simulink model "OFDM_64QAM_R14"  (Simulink 10.0)
settings: Solver=VariableStepDiscrete  StartTime=0.0  StopTime=5000  RelTol=1e-3  EnableMultiTasking=on
undefined symbols (not defined in the file): get
libraries: commutil2 x4, commsink2 x3, commdigbbndam2 x2, dspxfrm3 x2, dspindex x2, dspbuff3 x2, dspsnks4 x2, commchan2 x1, commrandsrc2 x1, dspobslib x1, simulink x1
settings Model: Creator=khanm  LastModifiedBy=bhisma
settings DataIOCC: ExternalInput=input_data  LimitDataPoints=on  SignalLoggingSaveFormat=ModelDataLogs  SaveOutput=off  SignalLogging=off  SaveTime=off
settings OptimizationCC: ExpressionDepthLimit=2147483647  InitFltsAndDblsToZero=on
settings DebuggingCC: SaveWithParameterizedLinksMsg=none  SignalResolutionControl=TryResolveAllWithWarning  MultiTaskDSMMsg=warning  MultiTaskCondExecSysMsg=none  FcnCallInpInsideContextMsg=warning  StateNameClashWarn=warning
settings SFSimCC: SimUseLocalCustomCode=on  CustomCodeUndefinedFunction=FilterOut
settings RTWCC: RTWUseLocalCustomCode=on
settings GRTTargetCC: TargetFcnLib=ansi_tfl_tmw.mat

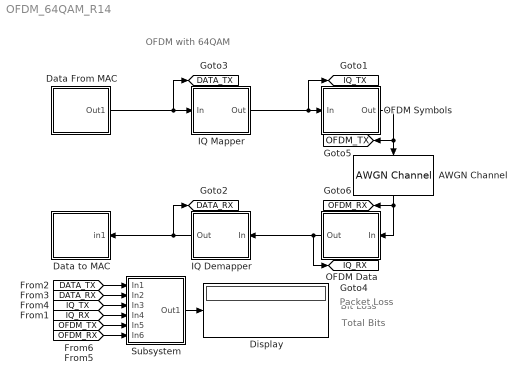
== system OFDM_64QAM_R14 ==
  note: OFDM with 64QAM
  note: Total Bits
  note: Bit Loss
  note: Packet Loss
  AWGN Channel : commchan2/AWGN Channel  SystemSampleTime=-1  seed=1  noiseMode="Signal to noise ratio  (SNR)"  EbNodB=10  EsNodB=40  SNRdB=60  bitsPerSym=2  Ps=0.01  Tsym=4e-6/80  variance=1
      settings: SourceProductName=Communications Toolbox  SourceProductBaseCode=CM
  Data From MAC : Subsystem
      mask Display: disp('Data Source');
  Data to MAC : Subsystem
      mask Display: disp('Data Sink');
  Display : Display
  IQ Demapper : Subsystem
      mask Display: disp('IQ Demapper');
  IQ Mapper : Subsystem
      mask Display: disp('IQ Mapper');
  OFDM Data : Subsystem
      mask Display: disp('OFDM \n Demodulator');
  OFDM Symbols : Subsystem
      mask Display: disp(' OFDM \n Modulation');
  Subsystem : Subsystem
      mask Display: disp('System\nPerformance\nTests');
  tag scope: DATA_RX=global, DATA_TX=global, IQ_RX=global, IQ_TX=global, OFDM_RX=global, OFDM_TX=global
  wires:
  IQ Demapper/1(Out) -> Data to MAC/1(in1), [DATA_RX]
  AWGN Channel/1 -> OFDM Data/1(In), [OFDM_RX]
  OFDM Data/1(Out) -> IQ Demapper/1(In), [IQ_RX]
  OFDM Symbols/1(Out) -> AWGN Channel/1, [OFDM_TX]
  IQ Mapper/1(Out) -> OFDM Symbols/1(In), [IQ_TX]
  [DATA_TX] -> Subsystem/1(In1)
  [DATA_RX] -> Subsystem/2(In2)
  [IQ_TX] -> Subsystem/3(In3)
  [IQ_RX] -> Subsystem/4(In4)
  [OFDM_TX] -> Subsystem/5(In5)
  [OFDM_RX] -> Subsystem/6(In6)
  Subsystem/1(Out1) -> Display/1
  Data From MAC/1(Out1) -> IQ Mapper/1(In), [DATA_TX]

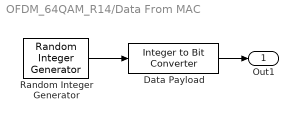
== system OFDM_64QAM_R14/Data From MAC ==
  Data Payload : commutil2/Integer to Bit Converter  nbits=6
      settings: SourceProductName=Communications Toolbox
  Random Integer Generator : commrandsrc2/Random Integer Generator  SystemSampleTime=-1  mul=32  seed=37  Ts=1/192  frameBased=on  sampPerFrame=192  orient=off
      settings: SourceProductName=Communications Toolbox  SourceProductBaseCode=CM
  Out1 : Outport
  wires:
  Random Integer Generator/1 -> Data Payload/1
  Data Payload/1 -> Out1/1

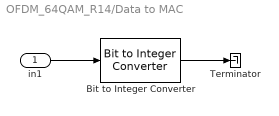
== system OFDM_64QAM_R14/Data to MAC ==
  in1 : Inport
  Bit to Integer Converter : commutil2/Bit to Integer Converter  nbits=6
      settings: SourceProductName=Communications Toolbox
  Terminator : Terminator
  wires:
  in1/1 -> Bit to Integer Converter/1
  Bit to Integer Converter/1 -> Terminator/1

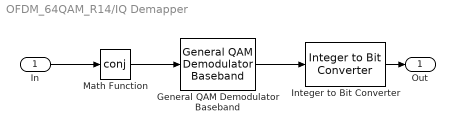
== system OFDM_64QAM_R14/IQ Demapper ==
  In : Inport
  General QAM Demodulator Baseband : commdigbbndam2/General QAM Demodulator Baseband  SigCon="[0.4629 + 0.4629i    0.4629 + 0.1543i    0.4629 + 0.7715i    0.4629 + 1.0801i    0.4629 - 0.4629i    0.4629 - 0.1543i    0.4629 - 0.7715i    0.4629 - 1.0801i    0.1543 + 0.4629i    0.1543 + 0.1543i    0.1543 + 0.7715i    0.1543 + 1.0801i    0.1543 - 0.4629i    0.1543 - 0.1543i    0.1543 - 0.7715i    0.1543 - 1.0801i    0.7715 + 0.4629i    0.7715 + 0.1543i    0.7715 + 0.7715i    0.7715 + 1.0801i    0.7715 - 0.4629i    0.7715 - 0.1543i    0.7715 - 0.7715i    0.7715 - 1.0801i    1.0801 + 0.4629i    1.0801 + 0.1543i    1.0801 + 0.7715i    1.0801 + 1.0801i    1.0801 - 0.4629i    1.0801 - 0.1543i    1.0801 - 0.7715i    1.0801 - 1.0801i   -0.4629 + 0.4629i   -0.4629 + 0.1543i   -0.4629 + 0.7715i   -0.4629 + 1.0801i   -0.4629 - 0.4629i   -0.4629 - 0.1543i   -0.4629 - 0.7715i   -0.4629 - 1.0801i   -0.1543 + 0.4629i   -0.1543 + 0.1543i   -0.1543 + 0.7715i   -0.1543 + 1.0801i   -0.1543 - 0.4629i   -0.1543 - 0.1543i   -0.1543 - 0.7715i   -0.1543 - 1.0801i   -0.7715 + 0.4629i   -0.7715 + 0.1543i   -0.7715 + 0.7715i   -0.7715 + 1.0801i   -0.7715 - 0.4629i   -0.7715 - 0.1543i   -0.7715 - 0.7715i   -0.7715 - 1.0801i   -1.0801 + 0.4629i   -1.0801 + 0.1543i   -1.0801 + 0.7715i   -1.0801 + 1.0801i   -1.0801 - 0.4629i   -1.0801 - 0.1543i   -1.0801 - 0.7715i   -1.0801 - 1.0801i]'"  numSamp=1
  Integer to Bit Converter : commutil2/Integer to Bit Converter  nbits=6
      settings: SourceProductName=Communications Toolbox
  Math Function : Math  Operator=conj  SaturateOnIntegerOverflow=on
  Out : Outport
  wires:
  General QAM Demodulator Baseband/1 -> Integer to Bit Converter/1
  In/1 -> Math Function/1
  Math Function/1 -> General QAM Demodulator Baseband/1
  Integer to Bit Converter/1 -> Out/1

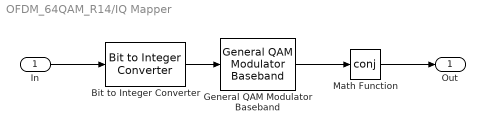
== system OFDM_64QAM_R14/IQ Mapper ==
  In : Inport
  Bit to Integer Converter : commutil2/Bit to Integer Converter  nbits=6
      settings: SourceProductName=Communications Toolbox
  General QAM Modulator Baseband : commdigbbndam2/General QAM Modulator Baseband  SigCon="[0.4629 + 0.4629i    0.4629 + 0.1543i    0.4629 + 0.7715i    0.4629 + 1.0801i    0.4629 - 0.4629i    0.4629 - 0.1543i    0.4629 - 0.7715i    0.4629 - 1.0801i    0.1543 + 0.4629i    0.1543 + 0.1543i    0.1543 + 0.7715i    0.1543 + 1.0801i    0.1543 - 0.4629i    0.1543 - 0.1543i    0.1543 - 0.7715i    0.1543 - 1.0801i    0.7715 + 0.4629i    0.7715 + 0.1543i    0.7715 + 0.7715i    0.7715 + 1.0801i    0.7715 - 0.4629i    0.7715 - 0.1543i    0.7715 - 0.7715i    0.7715 - 1.0801i    1.0801 + 0.4629i    1.0801 + 0.1543i    1.0801 + 0.7715i    1.0801 + 1.0801i    1.0801 - 0.4629i    1.0801 - 0.1543i    1.0801 - 0.7715i    1.0801 - 1.0801i   -0.4629 + 0.4629i   -0.4629 + 0.1543i   -0.4629 + 0.7715i   -0.4629 + 1.0801i   -0.4629 - 0.4629i   -0.4629 - 0.1543i   -0.4629 - 0.7715i   -0.4629 - 1.0801i   -0.1543 + 0.4629i   -0.1543 + 0.1543i   -0.1543 + 0.7715i   -0.1543 + 1.0801i   -0.1543 - 0.4629i   -0.1543 - 0.1543i   -0.1543 - 0.7715i   -0.1543 - 1.0801i   -0.7715 + 0.4629i   -0.7715 + 0.1543i   -0.7715 + 0.7715i   -0.7715 + 1.0801i   -0.7715 - 0.4629i   -0.7715 - 0.1543i   -0.7715 - 0.7715i   -0.7715 - 1.0801i   -1.0801 + 0.4629i   -1.0801 + 0.1543i   -1.0801 + 0.7715i   -1.0801 + 1.0801i   -1.0801 - 0.4629i   -1.0801 - 0.1543i   -1.0801 - 0.7715i   -1.0801 - 1.0801i]'"  numSamp=1
  Math Function : Math  Operator=conj  SaturateOnIntegerOverflow=on
  Out : Outport
  wires:
  In/1 -> Bit to Integer Converter/1
  General QAM Modulator Baseband/1 -> Math Function/1
  Math Function/1 -> Out/1
  Bit to Integer Converter/1 -> General QAM Modulator Baseband/1

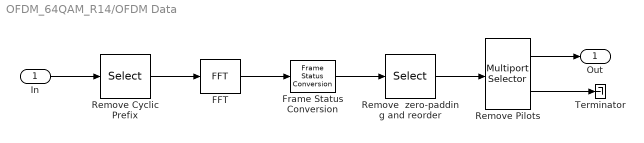
== system OFDM_64QAM_R14/OFDM Data ==
  In : Inport
  FFT : dspxfrm3/FFT  CompMethod=Table lookup  TableOpt=Speed  BitRevOrder=off  InheritFFTLength=on  FFTLength=64  SkipNorm=on  roundingMode=Floor  overflowMode=off
  Frame Status Conversion : dspobslib/Frame Status Conversion  SystemSampleTime=-1  growRefPort=off  outframe=Frame-based
      settings: SourceProductName=DSP System Toolbox  SourceProductBaseCode=DS
  Remove  zero-padding and reorder : Selector  InputPortWidth=256  IndexOptions=Index vector (dialog)  Indices=[29:128 130:229]  OutputSizes=[(-2)]
  Remove Pilots : dspindex/Multiport Selector  rowsOrCols=Rows  idxCellArray={[1:12 14:37 39:62 64:87 89:112 114:137 139:162 164:187 189:200],[13 38 63 88 113 138 163 188]}  idxErrMode=Clip Index
  Remove Cyclic Prefix : Selector  InputPortWidth=320  IndexOptions=Index vector (dialog)  Indices=[65:320]  OutputSizes=[(-2)]
  Terminator : Terminator
  Out : Outport
  wires:
  Frame Status Conversion/1 -> Remove  zero-padding and reorder/1
  FFT/1 -> Frame Status Conversion/1
  In/1 -> Remove Cyclic Prefix/1
  Remove  zero-padding and reorder/1 -> Remove Pilots/1
  Remove Pilots/1 -> Out/1
  Remove Pilots/2 -> Terminator/1
  Remove Cyclic Prefix/1 -> FFT/1

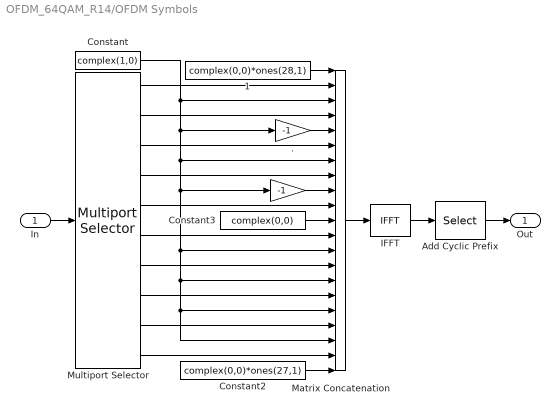
== system OFDM_64QAM_R14/OFDM Symbols ==
  In : Inport
  " " : Gain  Gain=-1
  " 1" : Constant  Value=complex(0,0)*ones(28,1)
  . : Gain  Gain=-1
  Add Cyclic Prefix : Selector  InputPortWidth=256  IndexOptions=Index vector (dialog)  Indices=[193:256 1:256]  OutputSizes=[(-2)]
  Constant : Constant  Value=complex(1,0)
  Constant2 : Constant  Value=complex(0,0)*ones(27,1)
  Constant3 : Constant  Value=complex(0,0)
  IFFT : dspxfrm3/IFFT  CompMethod=Table lookup  TableOpt=Speed  BitRevOrder=off  cs_in=off  SkipNorm=off  InheritFFTLength=on  FFTLength=64  mode=Complex  roundingMode=Floor  overflowMode=off
      settings: SourceProductName=DSP System Toolbox
  Matrix Concatenation : simulink/Math Operations/Matrix Concatenation  numInports=21  catMethod=Vertical
      settings: SourceProductName=Simulink  SourceProductBaseCode=SL
  Multiport Selector : dspindex/Multiport Selector  rowsOrCols=Rows  idxCellArray={1:12, 13:36, 37:60, 61:84, 85:96, 97:108, 109:132, 133:156, 157:180, 181:192}  idxErrMode=Clip Index
  Out : Outport
  wires:
  In/1 -> Multiport Selector/1
  Multiport Selector/9 -> Matrix Concatenation/18
  Multiport Selector/8 -> Matrix Concatenation/16
  Multiport Selector/7 -> Matrix Concatenation/14
  Multiport Selector/6 -> Matrix Concatenation/12
  Multiport Selector/5 -> Matrix Concatenation/10
  Multiport Selector/4 -> Matrix Concatenation/8
  Multiport Selector/3 -> Matrix Concatenation/6
  Multiport Selector/2 -> Matrix Concatenation/4
  Multiport Selector/1 -> Matrix Concatenation/2
  Multiport Selector/10 -> Matrix Concatenation/20
  Constant/1 -> Matrix Concatenation/3, Matrix Concatenation/7, " "/1, Matrix Concatenation/13, Matrix Concatenation/15, Matrix Concatenation/19, Matrix Concatenation/17, ./1
  " 1"/1 -> Matrix Concatenation/1
  Constant2/1 -> Matrix Concatenation/21
  ./1 -> Matrix Concatenation/5
  " "/1 -> Matrix Concatenation/9
  Constant3/1 -> Matrix Concatenation/11
  IFFT/1 -> Add Cyclic Prefix/1
  Matrix Concatenation/1 -> IFFT/1
  Add Cyclic Prefix/1 -> Out/1

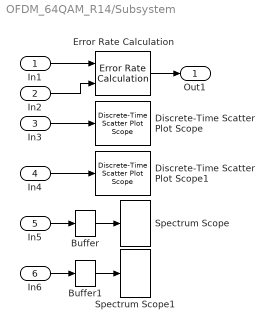
== system OFDM_64QAM_R14/Subsystem ==
  In1 : Inport
  In2 : Inport  Port=2
  In3 : Inport  Port=3
  In4 : Inport  Port=4
  In5 : Inport  Port=5
  In6 : Inport  Port=6
  Buffer : dspbuff3/Buffer  N=256  V=0  ic=0
      settings: SourceProductName=DSP System Toolbox  SourceProductBaseCode=DS
  Buffer1 : dspbuff3/Buffer  N=256  V=0  ic=0
      settings: SourceProductName=DSP System Toolbox  SourceProductBaseCode=DS
  Discrete-Time Scatter Plot Scope : commsink2/Discrete-Time Scatter Plot Scope  Tag=ScatterPlot  SystemSampleTime=-1  sampPerSymb=1  offsetEye=0  numTraces=64  numNewFrames=64  LineMarkers=.  LineColors=b  fading=on  render=on  AxisGrid=on  xMin=-0.572465428359361  xMax=1.80920677830553  yMin=-1.18813579470811  yMax=1.19353641195678  inphaseLabel=In-phase Amplitude  quadratureLabel=Quadrature Amplitude  openScopeAtSimStart=on  FrameNumber=off  FigPos=get(0,'defaultfigureposition');  figTitle=Scatter Plot  numLinesMax=8  block_type_=scatter
      settings: SourceProductName=Communications Toolbox  SourceProductBaseCode=CM
  Discrete-Time Scatter Plot Scope1 : commsink2/Discrete-Time Scatter Plot Scope  Tag=ScatterPlot  SystemSampleTime=-1  sampPerSymb=1  offsetEye=0  numTraces=64  numNewFrames=64  LineMarkers=.  LineColors=b  fading=on  render=on  AxisGrid=on  xMin=-0.572465430165662  xMax=1.80920678102707  yMin=-1.18813579747488  yMax=1.19353641371785  inphaseLabel=In-phase Amplitude  quadratureLabel=Quadrature Amplitude  openScopeAtSimStart=on  FrameNumber=off  FigPos=get(0,'defaultfigureposition');  figTitle=Scatter Plot  numLinesMax=8  block_type_=scatter
      settings: SourceProductName=Communications Toolbox  SourceProductBaseCode=CM
  Error Rate Calculation : commsink2/Error Rate Calculation  N=0  st_delay=0  cp_mode=Entire frame  subframe=[]  PMode=Port  WsName=grayBER  RsMode2=off  stop=on  numErr=1000000000  maxBits=10000000
      settings: SourceProductName=Communications Toolbox
  Spectrum Scope : dspsnks4/Spectrum Scope  SystemSampleTime=-1  ScopeProperties=on  Domain=Frequency  HorizSpan=1  UseBuffer=on  BufferSize=1024  Overlap=0  inpFftLenInherit=on  FFTlength=1024  numAvg=5  DisplayProperties=off  AxisGrid=off  Memory=off  FrameNumber=off  AxisLegend=off  AxisZoom=off  OpenScopeAtSimStart=on  OpenScopeImmediately=off  FigPos=get(0,'defaultfigureposition')  AxisProperties=off  XUnits=Hertz  XRange=[0...Fs/2]  InheritXIncr=on  XIncr=1.0  XLabel=Samples  XLimit=Auto  YUnits=dB  XMax=1  XMin=0  YLabel=Magnitude-squared, dB  LineProperties=off  wintypeSpecScope=Hann  RsSpecScope=50  betaSpecScope=5  winsampSpecScope=Periodic
      settings: SourceProductName=DSP System Toolbox  SourceProductBaseCode=DS  YMin=-49.5851620683178  YMax=-17.4535357375183
  Spectrum Scope1 : dspsnks4/Spectrum Scope  SystemSampleTime=-1  ScopeProperties=on  Domain=Frequency  HorizSpan=1  UseBuffer=on  BufferSize=1024  Overlap=0  inpFftLenInherit=on  FFTlength=1024  numAvg=5  DisplayProperties=off  AxisGrid=off  Memory=off  FrameNumber=off  AxisLegend=off  AxisZoom=off  OpenScopeAtSimStart=on  OpenScopeImmediately=off  FigPos=get(0,'defaultfigureposition')  AxisProperties=off  XUnits=Hertz  XRange=[0...Fs/2]  InheritXIncr=on  XIncr=1.0  XLabel=Samples  XLimit=Auto  YUnits=dB  XMax=1  XMin=0  YLabel=Magnitude-squared, dB  LineProperties=off  wintypeSpecScope=Hann  RsSpecScope=50  betaSpecScope=5  winsampSpecScope=Periodic
      settings: SourceProductName=DSP System Toolbox  SourceProductBaseCode=DS  YMin=-51.7490793915629  YMax=-17.1080597361603
  Out1 : Outport
  wires:
  Buffer1/1 -> Spectrum Scope1/1
  In1/1 -> Error Rate Calculation/1
  In2/1 -> Error Rate Calculation/2
  In5/1 -> Buffer/1
  Buffer/1 -> Spectrum Scope/1
  In6/1 -> Buffer1/1
  In3/1 -> Discrete-Time Scatter Plot Scope/1
  In4/1 -> Discrete-Time Scatter Plot Scope1/1
  Error Rate Calculation/1 -> Out1/1
